simulink model "MCC_Encoder"  (R2020b)
settings: Solver=VariableStepAuto  StartTime=0.0  StopTime=10.0  RelTol=1e-3
values from neighbouring files (symbols this model uses):
  deltaT = 0.01    [MCC_Encoder.m]
libraries: arduinolib x4
settings Model: Creator=xpess  LastModifiedBy=xpess

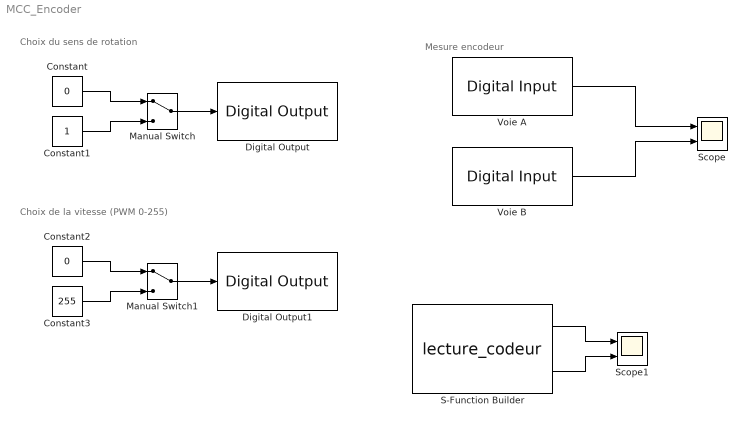
== system MCC_Encoder ==
  note: Choix du sens de rotation
  note: Choix de la vitesse (PWM 0-255)
  note: Mesure encodeur
  Constant : Constant  Value=0  SampleTime=deltaT
  Constant1 : Constant  SampleTime=deltaT
  Constant2 : Constant  Value=0  SampleTime=deltaT
  Constant3 : Constant  Value=255  SampleTime=deltaT
  Digital Output : arduinolib/Digital Output  pinNumber=9  Direction=output  blockPlatform=arduino
  Digital Output1 : arduinolib/Digital Output  pinNumber=9  Direction=output  blockPlatform=arduino
  Manual Switch : ManualSwitch
  Manual Switch1 : ManualSwitch
  S-Function Builder : S-Function  FunctionName=lecture_codeur  Parameters=boolean(1)  SFunctionModules=lecture_codeur_wrapper  SFunctionDeploymentMode=off  EnableBusSupport=off  mask(S-Function Builder){}
      mask help: Simulink:masks:SFunctionBuilder_MD
      mask init:
      | val = [[.9  0.75 0.75 1 1 .9 .9 1]',[1 1 0.75 0.75 .9 .9 1 .9]'];try , sys = get_param(gcb,'SfunBuilderFcnName');if isempty(sys), sys = get_param(gcb,'FunctionName'); end,catch, sys = get_param(gcb,'FunctionName'); end
      settings: CopyFcn=set_param(gcbh,'LinkStatus','none')  OpenFcn=sfunctionwizard(gcbh)
      mask Display:
      | plot(val(:,1),val(:,2))
      | disp(sys)
      | port_label('output',1,'compteur')
      | port_label('output',2,'omega')
  Scope : Scope  NumInputPorts=2
  Scope1 : Scope  NumInputPorts=2
  Voie A : arduinolib/Digital Input  pinNumber=8  mode=Default  Direction=input  SampleTime=0.1  blockPlatform=arduino
  Voie B : arduinolib/Digital Input  pinNumber=8  mode=Default  Direction=input  SampleTime=0.1  blockPlatform=arduino
  wires:
  Manual Switch/1 -> Digital Output/1
  Constant/1 -> Manual Switch/1
  Constant1/1 -> Manual Switch/2
  Constant3/1 -> Manual Switch1/2
  Manual Switch1/1 -> Digital Output1/1
  Constant2/1 -> Manual Switch1/1
  Voie A/1 -> Scope/1
  Voie B/1 -> Scope/2
  S-Function Builder/1 -> Scope1/1
  S-Function Builder/2 -> Scope1/2
